simulink model "lab_2"  (R2025a)
settings: Solver=VariableStepAuto  StartTime=0.0  StopTime=20  MaxStep=0.1  RelTol=1e-3
model workspace (MAT data in the model file):
  K = Simulink.Parameter
  K.Value = 2
  K.Complexity = 'real'
  K.Dimensions = [1 1]
  K.DataType = 'auto'
  T_3 = Simulink.Parameter
  T_3.Value = 0.1
  T_3.Complexity = 'real'
  T_3.Dimensions = [1 1]
  T_3.DataType = 'auto'
  T_4 = Simulink.Parameter
  T_4.Value = 0.3
  T_4.Complexity = 'real'
  T_4.Dimensions = [1 1]
  T_4.DataType = 'auto'
libraries: slctrl_linear x3
settings Model: Creator=konstantin  LastModifiedBy=konstantin

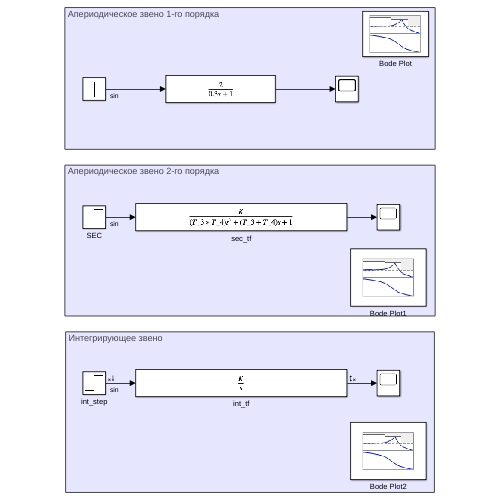
[thumbnail: Simulink's stored preview of the top-level diagram]
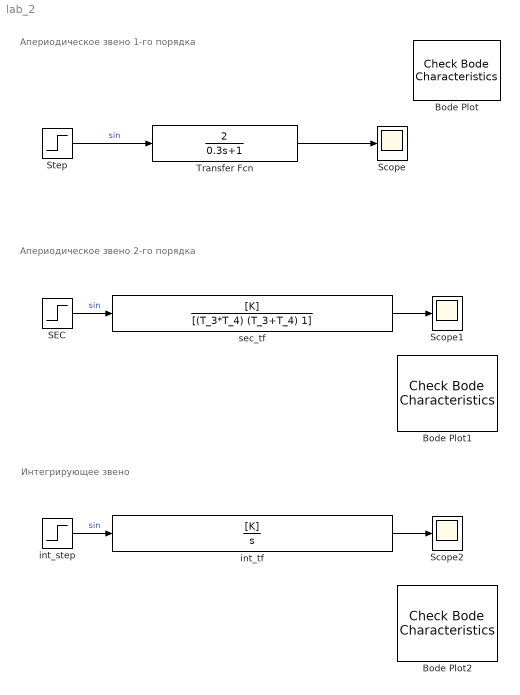
== system lab_2 ==
  note: Интегрирующее звено
  note: Апериодическое звено 2-го порядка
  note: Апериодическое звено 1-го порядка
  Bode Plot : slctrl_linear/Check Bode  Characteristics  InstantiateOnLoad=on  SaveOperatingPoints=off  LinearizationIOs={'/Step', 1, 'in', 'on', '';'/Transfer Fcn', 1, 'out', 'on', ''}  LinearizeAt=SnapshotTimes  SnapshotTimes=[0]  TriggerType=rising  SampleTime=auto  RateConversionMethod=zoh  PreWarpFreq=10  UseExactDelayModel=off  UseFullBlockNameLabels=off  UseBusSignalLabels=off  enabled=on  stopWhenAssertionFail=off  export=off  ViewDlgPos=[502 392 510 390]  OpenViewOnLoad=off  LaunchViewOnOpen=on  FrequencyUnits=Hz  MagnitudeUnits=dB  PhaseUnits=deg  TimeUnits=seconds  EnableUpperBound=off  UpperBoundFrequencies=[]  UpperBoundMagnitudes=[]  EnableLowerBound=off  LowerBoundFrequencies=[]  LowerBoundMagnitudes=[]
      settings: LibrarySourceBlock=slctrlblks/Linear Analysis Plots/Bode Plot  SaveToWorkspace=off  SaveName=sys
  Bode Plot1 : slctrl_linear/Check Bode  Characteristics  InstantiateOnLoad=on  SaveOperatingPoints=off  LinearizationIOs={'/SEC', 1, 'in', 'on', '';'/sec_tf', 1, 'out', 'on', ''}  LinearizeAt=SnapshotTimes  SnapshotTimes=[0]  TriggerType=rising  SampleTime=auto  RateConversionMethod=zoh  PreWarpFreq=10  UseExactDelayModel=off  UseFullBlockNameLabels=off  UseBusSignalLabels=off  enabled=on  stopWhenAssertionFail=off  export=off  ViewDlgPos=[1012 392 510 390]  OpenViewOnLoad=off  LaunchViewOnOpen=on  FrequencyUnits=Hz  MagnitudeUnits=dB  PhaseUnits=deg  TimeUnits=seconds  EnableUpperBound=off  UpperBoundFrequencies=[]  UpperBoundMagnitudes=[]  EnableLowerBound=off  LowerBoundFrequencies=[]  LowerBoundMagnitudes=[]
      settings: LibrarySourceBlock=slctrlblks/Linear Analysis Plots/Bode Plot  SaveToWorkspace=off  SaveName=sys
  Bode Plot2 : slctrl_linear/Check Bode  Characteristics  InstantiateOnLoad=on  SaveOperatingPoints=off  LinearizationIOs={'/int_step', 1, 'in', 'on', '';'/int_tf', 1, 'out', 'on', ''}  LinearizeAt=SnapshotTimes  SnapshotTimes=[0]  TriggerType=rising  SampleTime=auto  RateConversionMethod=zoh  PreWarpFreq=10  UseExactDelayModel=off  UseFullBlockNameLabels=off  UseBusSignalLabels=off  enabled=on  stopWhenAssertionFail=off  export=off  ViewDlgPos=[352 341 544 441]  OpenViewOnLoad=off  LaunchViewOnOpen=on  FrequencyUnits=Hz  MagnitudeUnits=dB  PhaseUnits=deg  TimeUnits=seconds  EnableUpperBound=off  UpperBoundFrequencies=[]  UpperBoundMagnitudes=[]  EnableLowerBound=off  LowerBoundFrequencies=[]  LowerBoundMagnitudes=[]
      settings: LibrarySourceBlock=slctrlblks/Linear Analysis Plots/Bode Plot  SaveToWorkspace=off  SaveName=sys
  SEC : Step  SampleTime=0
  Scope : Scope
      settings: ActiveDisplayYMinimum=-1.7797238236024764  ActiveDisplayYMaximum=1.8780138421904411
  Scope1 : Scope
      settings: ActiveDisplayYMinimum=-1.7797238236024764  ActiveDisplayYMaximum=1.8780138421904411
  Scope2 : Scope
      settings: ActiveDisplayYMinimum=-1.7797238236024764  ActiveDisplayYMaximum=1.8780138421904411  DataLoggingVariableName=ScopeData2
  Step : Step  SampleTime=0
  Transfer Fcn : TransferFcn  Numerator=[2]  Denominator=[0.3 1]
  int_step : Step  SampleTime=0
  int_tf : TransferFcn  Numerator=[K]  Denominator=[1 0]
  sec_tf : TransferFcn  Numerator=[K]  Denominator=[(T_3*T_4) (T_3+T_4) 1]
  wires:
  Step/1 -> Transfer Fcn/1  "sin"
  Transfer Fcn/1 -> Scope/1
  SEC/1 -> sec_tf/1  "sin"
  sec_tf/1 -> Scope1/1
  int_step/1 -> int_tf/1  "sin"
  int_tf/1 -> Scope2/1
